simulink model "GPI1"  (Simulink 7.0)
settings: Solver=ode45  StartTime=0.0  StopTime=1000.0  RelTol=1e-3
values from neighbouring files (symbols this model uses):
  A_gpegpi = 1    [data_GPE.m]    (also in data_GPI.m)
  A_gpi = 2    [data_GPI.m]
  A_stngpi = 1    [data_GPI.m]    (also in data_STN.m)
  B_gpegpi = .1    (= 0.1)    [data_GPE.m]    (also in data_GPI.m)
  B_gpi = .08    (= 0.08)    [data_GPI.m]
  B_stngpi = .05    (= 0.05)    [data_GPI.m]    (also in data_STN.m)
  c_gpi = 1    [data_GPI.m]
  cagi0 = i_v_16(289:304)    [launch_sysGPI_mod.m]
  egpegpi = -100    [data_synapses.m]
  ek_gpi = -80.0    (= -80)    [data_GPI.m]
  el_gpi = -55.0    (= -55)    [data_GPI.m]
  epsil_gpi = 1*10^-4    (= 0.0001)    [data_GPI.m]
  estngpi = 0    [data_synapses.m]
  gahp_gpi = 30.0    (= 30)    [data_GPI.m]
  gca_gpi = 0.15    [data_GPI.m]
  ggpegpi = ggpegpi_vec(i)    [CN_launch_CN_analyze_TAL2.m]    (also in data_synapses.m = 1; launch_sysGPI_mod.m = 0.3)
  gk_gpi = 30.0    (= 30)    [data_GPI.m]
  gl_gpi = .1    (= 0.1)    [data_GPI.m]
  gna_gpi = 120    [data_GPI.m]
  gstngpi = .3    (= 0.3)    [data_synapses.m]
  gt_gpi = .5    (= 0.5)    [data_GPI.m]
  hgi0 = i_v_16(241:256)    [launch_sysGPI_mod.m]
  k1_gpi = 30.0    (= 30)    [data_GPI.m]
  kca_gpi = 15    [data_GPI.m]
  ngi0 = i_v_16(257:272)    [launch_sysGPI_mod.m]
  phih_gpi = 0.05    [data_GPI.m]
  phin_gpi = 0.1    [data_GPI.m]
  phir_gpi = 1    [data_GPI.m]
  rgi0 = i_v_16(273:288)    [launch_sysGPI_mod.m]
  sgi0 = i_v_16(305:320)    [launch_sysGPI_mod.m]
  sig0 = i_v_16(209:224)    [launch_sysGPI_mod.m]
  sigmaa_gpi = 2    [data_GPI.m]
  sigmagh_gpe = 2.0    (= 2)    [data_GPE.m]
  sigmagh_gpi = 2.0    (= 2)    [data_GPI.m]
  sigmagh_stn = 8.0    (= 8)    [data_STN.m]
  sigmah_gpi = -12    [data_GPI.m]
  sigmam_gpi = 10.0    (= 10)    [data_GPI.m]
  sigman_gpi = 14.0    (= 14)    [data_GPI.m]
  sigmar_gpi = -2.0    (= -2)    [data_GPI.m]
  sigmas_gpi = 2    [data_GPI.m]
  sigmatauh_gpi = -12    [data_GPI.m]
  sigmataun_gpi = -12.0    (= -12)    [data_GPI.m]
  sis0 = i_v_16(97:112)    [launch_sysGPI_mod.m]
  tauh0_gpi = .05    (= 0.05)    [data_GPI.m]
  tauh1_gpi = .27    (= 0.27)    [data_GPI.m]
  taun0_gpi = .05    (= 0.05)    [data_GPI.m]
  taun1_gpi = .27    (= 0.27)    [data_GPI.m]
  taur_gpi = 30.0    (= 30)    [data_GPI.m]
  theta_gpe = 20    [data_GPE.m]    (also in data_GPI.m)
  theta_gpi = 20    [data_GPI.m]
  theta_stn = 30    [data_GPI.m]    (also in data_STN.m)
  thetaa_gpi = -57.0    (= -57)    [data_GPI.m]
  thetagh_gpe = -57.0    (= -57)    [data_GPE.m]
  thetagh_gpi = -57.0    (= -57)    [data_GPI.m]
  thetagh_stn = -39.0    (= -39)    [data_STN.m]
  thetah_gpi = -58.0    (= -58)    [data_GPI.m]
  thetam_gpi = -37.0    (= -37)    [data_GPI.m]
  thetan_gpi = -50.0    (= -50)    [data_GPI.m]
  thetar_gpi = -70.0    (= -70)    [data_GPI.m]
  thetas_gpi = -35.0    (= -35)    [data_GPI.m]
  thetatauh_gpi = -40.0    (= -40)    [data_GPI.m]
  thetataun_gpi = -40.0    (= -40)    [data_GPI.m]
  vgi0 = i_v_16(225:240)    [launch_sysGPI_mod.m]
(part 1 of 6)
settings Model: Creator=marco  LastModifiedBy=marco  ExtModeAutoUpdateStatusClock=off
settings DataIOCC: ExternalInput=[t1,u1]  LoadExternalInput=on  SaveOutput=off  SignalLogging=off  SaveTime=off  SignalLoggingName=sigsOut
settings OptimizationCC: BooleanDataType=off
settings DebuggingCC: SaveWithParameterizedLinksMsg=none  SignalResolutionControl=TryResolveAllWithWarning  SolverPrmCheckMsg=none  MultiTaskDSMMsg=warning  MultiTaskCondExecSysMsg=none  StrictBusMsg=None
settings HardwareCC: TargetUnknown=on
settings RTWCC: IncludeERTFirstTime=on
settings GRTTargetCC: TargetFcnLib=ansi_tfl_tmw.mat

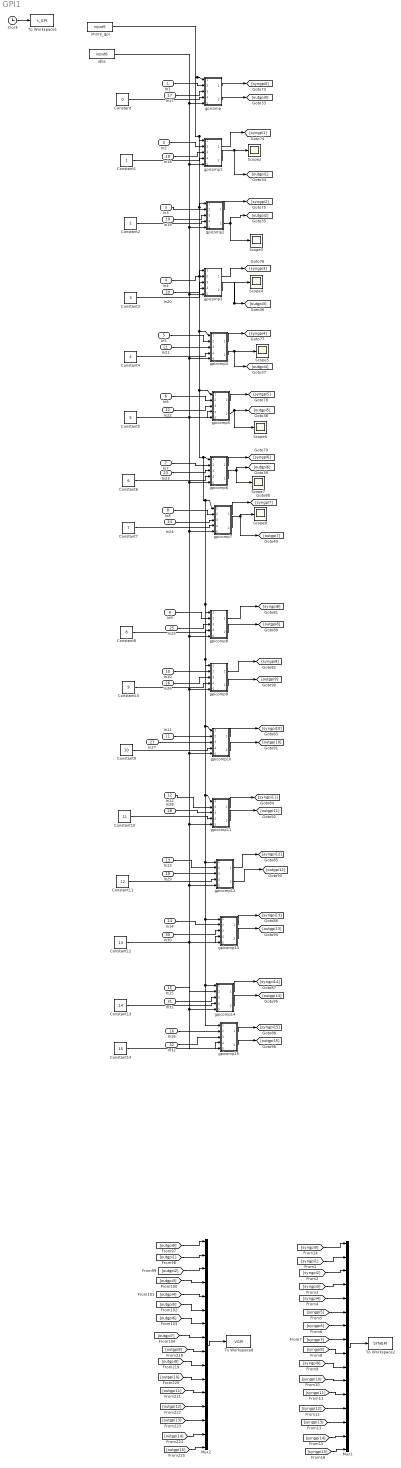
== system GPI1 ==
  In1 : Inport  OutDataType=sfix(16)  OutScaling=2^0
  In2 : Inport  Port=2  OutDataType=sfix(16)  OutScaling=2^0
  In3 : Inport  Port=3  OutDataType=sfix(16)  OutScaling=2^0
  In4 : Inport  Port=4  OutDataType=sfix(16)  OutScaling=2^0
  In5 : Inport  Port=5  OutDataType=sfix(16)  OutScaling=2^0
  In6 : Inport  Port=6  OutDataType=sfix(16)  OutScaling=2^0
  In7 : Inport  Port=7  OutDataType=sfix(16)  OutScaling=2^0
  In8 : Inport  Port=8  OutDataType=sfix(16)  OutScaling=2^0
  In9 : Inport  Port=9  OutDataType=sfix(16)  OutScaling=2^0
  In10 : Inport  Port=10  OutDataType=sfix(16)  OutScaling=2^0
  In11 : Inport  Port=11  OutDataType=sfix(16)  OutScaling=2^0
  In12 : Inport  Port=12  OutDataType=sfix(16)  OutScaling=2^0
  In13 : Inport  Port=13  OutDataType=sfix(16)  OutScaling=2^0
  In14 : Inport  Port=14  OutDataType=sfix(16)  OutScaling=2^0
  In15 : Inport  Port=15  OutDataType=sfix(16)  OutScaling=2^0
  In16 : Inport  Port=16  OutDataType=sfix(16)  OutScaling=2^0
  In17 : Inport  Port=17  OutDataType=sfix(16)  OutScaling=2^0
  In18 : Inport  Port=18  OutDataType=sfix(16)  OutScaling=2^0
  In19 : Inport  Port=19  OutDataType=sfix(16)  OutScaling=2^0
  In20 : Inport  Port=20  OutDataType=sfix(16)  OutScaling=2^0
  In21 : Inport  Port=21  OutDataType=sfix(16)  OutScaling=2^0
  In22 : Inport  Port=22  OutDataType=sfix(16)  OutScaling=2^0
  In23 : Inport  Port=23  OutDataType=sfix(16)  OutScaling=2^0
  In24 : Inport  Port=24  OutDataType=sfix(16)  OutScaling=2^0
  In25 : Inport  Port=25  OutDataType=sfix(16)  OutScaling=2^0
  In26 : Inport  Port=26  OutDataType=sfix(16)  OutScaling=2^0
  In27 : Inport  Port=27  OutDataType=sfix(16)  OutScaling=2^0
  In28 : Inport  Port=28  OutDataType=sfix(16)  OutScaling=2^0
  In29 : Inport  Port=29  OutDataType=sfix(16)  OutScaling=2^0
  In30 : Inport  Port=30  OutDataType=sfix(16)  OutScaling=2^0
  In31 : Inport  Port=31  OutDataType=sfix(16)  OutScaling=2^0
  In32 : Inport  Port=32  OutDataType=sfix(16)  OutScaling=2^0
  Clock : Clock
      settings: Decimation=10
  Constant : Constant  Value=0  OutDataType=sfix(16)  OutScaling=2^0
  Constant1 : Constant  OutDataType=sfix(16)  OutScaling=2^0
  Constant10 : Constant  Value=11  OutDataType=sfix(16)  OutScaling=2^0
  Constant11 : Constant  Value=12  OutDataType=sfix(16)  OutScaling=2^0
  Constant12 : Constant  Value=13  OutDataType=sfix(16)  OutScaling=2^0
  Constant13 : Constant  Value=14  OutDataType=sfix(16)  OutScaling=2^0
  Constant14 : Constant  Value=15  OutDataType=sfix(16)  OutScaling=2^0
  Constant15 : Constant  Value=9  OutDataType=sfix(16)  OutScaling=2^0
  Constant2 : Constant  Value=2  OutDataType=sfix(16)  OutScaling=2^0
  Constant3 : Constant  Value=3  OutDataType=sfix(16)  OutScaling=2^0
  Constant4 : Constant  Value=4  OutDataType=sfix(16)  OutScaling=2^0
  Constant5 : Constant  Value=5  OutDataType=sfix(16)  OutScaling=2^0
  Constant6 : Constant  Value=6  OutDataType=sfix(16)  OutScaling=2^0
  Constant7 : Constant  Value=7  OutDataType=sfix(16)  OutScaling=2^0
  Constant8 : Constant  Value=8  OutDataType=sfix(16)  OutScaling=2^0
  Constant9 : Constant  Value=10  OutDataType=sfix(16)  OutScaling=2^0
  Mux1 : Mux  Inputs=16
  Mux2 : Mux  Inputs=16
  Scope{2..8} (7 alike) : Scope
      Scope2 settings: YMin=-90  YMax=60  SaveName=ScopeData2
      Scope3 settings: YMin=-90  YMax=60  SaveName=ScopeData3
      Scope4 settings: YMin=-90  YMax=60  SaveName=ScopeData4
      Scope5 settings: SaveName=ScopeData5
      Scope6 settings: YMin=-90  YMax=60  SaveName=ScopeData6
      Scope7 settings: SaveName=ScopeData7
      Scope8 settings: YMin=-90  YMax=60  SaveName=ScopeData8
  To Workspace1 : ToWorkspace  VariableName=t_GPI  SampleTime=-1  SaveFormat=Array
  To Workspace2 : ToWorkspace  VariableName=SYNGPI  SampleTime=-1  SaveFormat=Array
  To Workspace8 : ToWorkspace  VariableName=VGPI  SampleTime=-1  SaveFormat=Array
  gpicomp : Subsystem
  gpicomp1 : Subsystem
  gpicomp10 : Subsystem
  gpicomp11 : Subsystem
  gpicomp12 : Subsystem
  gpicomp13 : Subsystem
  gpicomp14 : Subsystem
  gpicomp15 : Subsystem
  gpicomp2 : Subsystem
  gpicomp3 : Subsystem
  gpicomp4 : Subsystem
  gpicomp5 : Subsystem
  gpicomp6 : Subsystem
  gpicomp7 : Subsystem
  gpicomp8 : Subsystem
  gpicomp9 : Subsystem
  idbs : FromWorkspace  VariableName=input6  SampleTime=0.01
  imore_gpi : FromWorkspace  VariableName=input5  SampleTime=1
  wires:
  Clock/1 -> To Workspace1/1
  gpicomp6/2(Out2) -> Scope7/1, [outgpi6]
  gpicomp5/2(Out2) -> Scope6/1, [outgpi5]
  gpicomp4/2(Out2) -> Scope5/1, [outgpi4]
  gpicomp3/2(Out2) -> Scope4/1, [outgpi3]
  gpicomp/2(Out2) -> [outgpi0]
  gpicomp2/2(Out2) -> Scope3/1, [outgpi2]
  gpicomp1/2(Out2) -> Scope2/1, [outgpi1]
  imore_gpi/1 -> gpicomp/1(In1), gpicomp14/1(In1), gpicomp15/1(In1), gpicomp13/1(In1), gpicomp12/1(In1), gpicomp11/1(In1), gpicomp10/1(In1), gpicomp9/1(In1), gpicomp8/1(In1), gpicomp7/1(In1), gpicomp6/1(In1), gpicomp5/1(In1), gpicomp4/1(In1), gpicomp3/1(In1), gpicomp2/1(In1), gpicomp1/1(In1)
  gpicomp7/2(Out2) -> Scope8/1, [outgpi7]
  [outgpi0] -> Mux2/1
  [outgpi1] -> Mux2/2
  [outgpi2] -> Mux2/3
  [outgpi3] -> Mux2/4
  [outgpi4] -> Mux2/5
  [outgpi5] -> Mux2/6
  [outgpi6] -> Mux2/7
  [outgpi7] -> Mux2/8
  Mux2/1 -> To Workspace8/1
  gpicomp/1(Out1) -> [syngpi0]
  gpicomp1/1(Out1) -> [syngpi1]
  gpicomp2/1(Out1) -> [syngpi2]
  gpicomp3/1(Out1) -> [syngpi3]
  gpicomp4/1(Out1) -> [syngpi4]
  gpicomp5/1(Out1) -> [syngpi5]
  gpicomp6/1(Out1) -> [syngpi6]
  gpicomp7/1(Out1) -> [syngpi7]
  gpicomp8/1(Out1) -> [syngpi8]
  gpicomp9/1(Out1) -> [syngpi9]
  gpicomp10/1(Out1) -> [syngpi10]
  gpicomp11/1(Out1) -> [syngpi11]
  gpicomp12/1(Out1) -> [syngpi12]
  gpicomp13/1(Out1) -> [syngpi13]
  gpicomp14/1(Out1) -> [syngpi14]
  gpicomp15/1(Out1) -> [syngpi15]
  gpicomp13/2(Out2) -> [outgpi13]
  gpicomp14/2(Out2) -> [outgpi14]
  gpicomp15/2(Out2) -> [outgpi15]
  gpicomp12/2(Out2) -> [outgpi12]
  gpicomp11/2(Out2) -> [outgpi11]
  gpicomp10/2(Out2) -> [outgpi10]
  gpicomp9/2(Out2) -> [outgpi9]
  gpicomp8/2(Out2) -> [outgpi8]
  [outgpi8] -> Mux2/9
  [outgpi9] -> Mux2/10
  [outgpi10] -> Mux2/11
  [outgpi11] -> Mux2/12
  [outgpi12] -> Mux2/13
  [outgpi13] -> Mux2/14
  [outgpi14] -> Mux2/15
  [outgpi15] -> Mux2/16
  Constant14/1 -> gpicomp15/4(In4)
  Constant13/1 -> gpicomp14/4(In4)
  Constant12/1 -> gpicomp13/4(In4)
  Constant11/1 -> gpicomp12/4(In4)
  Constant10/1 -> gpicomp11/4(In4)
  Constant9/1 -> gpicomp10/4(In4)
  Constant15/1 -> gpicomp9/4(In4)
  Constant8/1 -> gpicomp8/4(In4)
  Constant7/1 -> gpicomp7/4(In4)
  Constant6/1 -> gpicomp6/4(In4)
  Constant5/1 -> gpicomp5/4(In4)
  Constant4/1 -> gpicomp4/4(In4)
  Constant3/1 -> gpicomp3/4(In4)
  Constant2/1 -> gpicomp2/4(In4)
  Constant1/1 -> gpicomp1/4(In4)
  Constant/1 -> gpicomp/4(In4)
  In1/1 -> gpicomp/2(In2)
  In2/1 -> gpicomp1/2(In2)
  In3/1 -> gpicomp2/2(In2)
  In4/1 -> gpicomp3/2(In2)
  In5/1 -> gpicomp4/2(In2)
  In6/1 -> gpicomp5/2(In2)
  In7/1 -> gpicomp6/2(In2)
  In8/1 -> gpicomp7/2(In2)
  In9/1 -> gpicomp8/2(In2)
  In10/1 -> gpicomp9/2(In2)
  In11/1 -> gpicomp10/2(In2)
  In12/1 -> gpicomp11/2(In2)
  In13/1 -> gpicomp12/2(In2)
  In14/1 -> gpicomp13/2(In2)
  In15/1 -> gpicomp14/2(In2)
  In16/1 -> gpicomp15/2(In2)
  In32/1 -> gpicomp15/3(In3)
  In31/1 -> gpicomp14/3(In3)
  In30/1 -> gpicomp13/3(In3)
  In29/1 -> gpicomp12/3(In3)
  In28/1 -> gpicomp11/3(In3)
  In27/1 -> gpicomp10/3(In3)
  In26/1 -> gpicomp9/3(In3)
  In25/1 -> gpicomp8/3(In3)
  In24/1 -> gpicomp7/3(In3)
  In23/1 -> gpicomp6/3(In3)
  In22/1 -> gpicomp5/3(In3)
  In21/1 -> gpicomp4/3(In3)
  In20/1 -> gpicomp3/3(In3)
  In19/1 -> gpicomp2/3(In3)
  In18/1 -> gpicomp1/3(In3)
  In17/1 -> gpicomp/3(In3)
  [syngpi0] -> Mux1/1
  [syngpi2] -> Mux1/3
  Mux1/1 -> To Workspace2/1
  [syngpi8] -> Mux1/9
  [syngpi9] -> Mux1/10
  [syngpi10] -> Mux1/11
  [syngpi11] -> Mux1/12
  [syngpi12] -> Mux1/13
  [syngpi13] -> Mux1/14
  [syngpi14] -> Mux1/15
  [syngpi15] -> Mux1/16
  [syngpi1] -> Mux1/2
  [syngpi3] -> Mux1/4
  [syngpi4] -> Mux1/5
  [syngpi5] -> Mux1/6
  [syngpi6] -> Mux1/7
  [syngpi7] -> Mux1/8
  idbs/1 -> gpicomp/5(In5), gpicomp1/5(In5), gpicomp2/5(In5), gpicomp3/5(In5), gpicomp4/5(In5), gpicomp6/5(In5), gpicomp7/5(In5), gpicomp8/5(In5), gpicomp9/5(In5), gpicomp10/5(In5), gpicomp11/5(In5), gpicomp12/5(In5), gpicomp14/5(In5), gpicomp15/5(In5), gpicomp13/5(In5), gpicomp5/5(In5)

== system GPI1/gpicomp ==
  In1 : Inport  OutDataType=sfix(16)  OutScaling=2^0
  In2 : Inport  Port=2  OutDataType=sfix(16)  OutScaling=2^0
  In3 : Inport  Port=3  OutDataType=sfix(16)  OutScaling=2^0
  In4 : Inport  Port=4  OutDataType=sfix(16)  OutScaling=2^0
  In5 : Inport  Port=5  OutDataType=sfix(16)  OutScaling=2^0
  Constant : Constant  Value=sis0  OutDataType=sfix(16)  OutScaling=2^0
  Constant1 : Constant  Value=sig0  OutDataType=sfix(16)  OutScaling=2^0
  Constant2 : Constant  Value=sgi0  OutDataType=sfix(16)  OutScaling=2^0
  Selector1 : Selector  IndexMode=Zero-based  IndexOptions=Index vector (port)  Indices=[1 3]  OutputSizes=1
  Selector2 : Selector  IndexMode=Zero-based  IndexOptions=Index vector (port)  Indices=[1 3]  OutputSizes=1
  Selector5 : Selector  IndexMode=Zero-based  IndexOptions=Index vector (port)  Indices=[1 3]  OutputSizes=1
  gpi_cell : Subsystem
  igpegpi : Subsystem
  istngpi : Subsystem
  syn_gpegpi : Subsystem
  syn_gpegpi1 : Subsystem
  syn_stngpi : Subsystem
  Out1 : Outport  OutDataType=sfix(16)  OutScaling=2^0
  Out2 : Outport  Port=2  OutDataType=sfix(16)  OutScaling=2^0
  wires:
  igpegpi/1(Out1) -> gpi_cell/3(In3)
  istngpi/1(Out1) -> gpi_cell/2(In2)
  syn_gpegpi/1(Out1) -> igpegpi/1(In1)
  syn_stngpi/1(Out1) -> istngpi/1(In1)
  syn_gpegpi1/1(Out1) -> Out1/1
  In1/1 -> gpi_cell/1(In1)
  In2/1 -> syn_stngpi/1(In1)
  In3/1 -> syn_gpegpi/1(In1)
  gpi_cell/1(Out1) -> Out2/1, istngpi/2(In3), igpegpi/2(In3), syn_gpegpi1/1(In1)
  Selector2/1 -> syn_gpegpi1/2(In2)
  In4/1 -> Selector5/2, Selector2/2, gpi_cell/4(In4), Selector1/2
  Selector5/1 -> syn_stngpi/2(In2)
  Selector1/1 -> syn_gpegpi/2(In2)
  Constant2/1 -> Selector2/1
  Constant/1 -> Selector5/1
  Constant1/1 -> Selector1/1
  In5/1 -> gpi_cell/5(In5)

== system GPI1/gpicomp1 ==
  In1 : Inport  OutDataType=sfix(16)  OutScaling=2^0
  In2 : Inport  Port=2  OutDataType=sfix(16)  OutScaling=2^0
  In3 : Inport  Port=3  OutDataType=sfix(16)  OutScaling=2^0
  In4 : Inport  Port=4  OutDataType=sfix(16)  OutScaling=2^0
  In5 : Inport  Port=5  OutDataType=sfix(16)  OutScaling=2^0
  Constant : Constant  Value=sis0  OutDataType=sfix(16)  OutScaling=2^0
  Constant1 : Constant  Value=sig0  OutDataType=sfix(16)  OutScaling=2^0
  Constant2 : Constant  Value=sgi0  OutDataType=sfix(16)  OutScaling=2^0
  Selector1 : Selector  IndexMode=Zero-based  IndexOptions=Index vector (port)  Indices=[1 3]  OutputSizes=1
  Selector2 : Selector  IndexMode=Zero-based  IndexOptions=Index vector (port)  Indices=[1 3]  OutputSizes=1
  Selector5 : Selector  IndexMode=Zero-based  IndexOptions=Index vector (port)  Indices=[1 3]  OutputSizes=1
  gpi_cell : Subsystem
  igpegpi : Subsystem
  istngpi : Subsystem
  syn_gpegpi : Subsystem
  syn_gpegpi1 : Subsystem
  syn_stngpi : Subsystem
  Out1 : Outport  OutDataType=sfix(16)  OutScaling=2^0
  Out2 : Outport  Port=2  OutDataType=sfix(16)  OutScaling=2^0
  wires:
  igpegpi/1(Out1) -> gpi_cell/3(In3)
  istngpi/1(Out1) -> gpi_cell/2(In2)
  syn_gpegpi/1(Out1) -> igpegpi/1(In1)
  syn_stngpi/1(Out1) -> istngpi/1(In1)
  syn_gpegpi1/1(Out1) -> Out1/1
  In1/1 -> gpi_cell/1(In1)
  In2/1 -> syn_stngpi/1(In1)
  In3/1 -> syn_gpegpi/1(In1)
  gpi_cell/1(Out1) -> Out2/1, istngpi/2(In3), igpegpi/2(In3), syn_gpegpi1/1(In1)
  Selector2/1 -> syn_gpegpi1/2(In2)
  In4/1 -> Selector5/2, Selector2/2, gpi_cell/4(In4), Selector1/2
  Selector5/1 -> syn_stngpi/2(In2)
  Selector1/1 -> syn_gpegpi/2(In2)
  Constant2/1 -> Selector2/1
  Constant/1 -> Selector5/1
  Constant1/1 -> Selector1/1
  In5/1 -> gpi_cell/5(In5)

== system GPI1/gpicomp10 ==
  In1 : Inport  OutDataType=sfix(16)  OutScaling=2^0
  In2 : Inport  Port=2  OutDataType=sfix(16)  OutScaling=2^0
  In3 : Inport  Port=3  OutDataType=sfix(16)  OutScaling=2^0
  In4 : Inport  Port=4  OutDataType=sfix(16)  OutScaling=2^0
  In5 : Inport  Port=5  OutDataType=sfix(16)  OutScaling=2^0
  Constant : Constant  Value=sis0  OutDataType=sfix(16)  OutScaling=2^0
  Constant1 : Constant  Value=sig0  OutDataType=sfix(16)  OutScaling=2^0
  Constant2 : Constant  Value=sgi0  OutDataType=sfix(16)  OutScaling=2^0
  Selector1 : Selector  IndexMode=Zero-based  IndexOptions=Index vector (port)  Indices=[1 3]  OutputSizes=1
  Selector2 : Selector  IndexMode=Zero-based  IndexOptions=Index vector (port)  Indices=[1 3]  OutputSizes=1
  Selector5 : Selector  IndexMode=Zero-based  IndexOptions=Index vector (port)  Indices=[1 3]  OutputSizes=1
  gpi_cell : Subsystem
  igpegpi : Subsystem
  istngpi : Subsystem
  syn_gpegpi : Subsystem
  syn_gpegpi1 : Subsystem
  syn_stngpi : Subsystem
  Out1 : Outport  OutDataType=sfix(16)  OutScaling=2^0
  Out2 : Outport  Port=2  OutDataType=sfix(16)  OutScaling=2^0
  wires:
  igpegpi/1(Out1) -> gpi_cell/3(In3)
  istngpi/1(Out1) -> gpi_cell/2(In2)
  syn_gpegpi/1(Out1) -> igpegpi/1(In1)
  syn_stngpi/1(Out1) -> istngpi/1(In1)
  syn_gpegpi1/1(Out1) -> Out1/1
  In1/1 -> gpi_cell/1(In1)
  In2/1 -> syn_stngpi/1(In1)
  In3/1 -> syn_gpegpi/1(In1)
  gpi_cell/1(Out1) -> Out2/1, istngpi/2(In3), igpegpi/2(In3), syn_gpegpi1/1(In1)
  Selector2/1 -> syn_gpegpi1/2(In2)
  In4/1 -> Selector5/2, Selector2/2, gpi_cell/4(In4), Selector1/2
  Selector5/1 -> syn_stngpi/2(In2)
  Selector1/1 -> syn_gpegpi/2(In2)
  Constant2/1 -> Selector2/1
  Constant/1 -> Selector5/1
  Constant1/1 -> Selector1/1
  In5/1 -> gpi_cell/5(In5)

== system GPI1/gpicomp11 ==
  In1 : Inport  OutDataType=sfix(16)  OutScaling=2^0
  In2 : Inport  Port=2  OutDataType=sfix(16)  OutScaling=2^0
  In3 : Inport  Port=3  OutDataType=sfix(16)  OutScaling=2^0
  In4 : Inport  Port=4  OutDataType=sfix(16)  OutScaling=2^0
  In5 : Inport  Port=5  OutDataType=sfix(16)  OutScaling=2^0
  Constant : Constant  Value=sis0  OutDataType=sfix(16)  OutScaling=2^0
  Constant1 : Constant  Value=sig0  OutDataType=sfix(16)  OutScaling=2^0
  Constant2 : Constant  Value=sgi0  OutDataType=sfix(16)  OutScaling=2^0
  Selector1 : Selector  IndexMode=Zero-based  IndexOptions=Index vector (port)  Indices=[1 3]  OutputSizes=1
  Selector2 : Selector  IndexMode=Zero-based  IndexOptions=Index vector (port)  Indices=[1 3]  OutputSizes=1
  Selector5 : Selector  IndexMode=Zero-based  IndexOptions=Index vector (port)  Indices=[1 3]  OutputSizes=1
  gpi_cell : Subsystem
  igpegpi : Subsystem
  istngpi : Subsystem
  syn_gpegpi : Subsystem
  syn_gpegpi1 : Subsystem
  syn_stngpi : Subsystem
  Out1 : Outport  OutDataType=sfix(16)  OutScaling=2^0
  Out2 : Outport  Port=2  OutDataType=sfix(16)  OutScaling=2^0
  wires:
  igpegpi/1(Out1) -> gpi_cell/3(In3)
  istngpi/1(Out1) -> gpi_cell/2(In2)
  syn_gpegpi/1(Out1) -> igpegpi/1(In1)
  syn_stngpi/1(Out1) -> istngpi/1(In1)
  syn_gpegpi1/1(Out1) -> Out1/1
  In1/1 -> gpi_cell/1(In1)
  In2/1 -> syn_stngpi/1(In1)
  In3/1 -> syn_gpegpi/1(In1)
  gpi_cell/1(Out1) -> Out2/1, istngpi/2(In3), igpegpi/2(In3), syn_gpegpi1/1(In1)
  Selector2/1 -> syn_gpegpi1/2(In2)
  In4/1 -> Selector5/2, Selector2/2, gpi_cell/4(In4), Selector1/2
  Selector5/1 -> syn_stngpi/2(In2)
  Selector1/1 -> syn_gpegpi/2(In2)
  Constant2/1 -> Selector2/1
  Constant/1 -> Selector5/1
  Constant1/1 -> Selector1/1
  In5/1 -> gpi_cell/5(In5)

== system GPI1/gpicomp12 ==
  In1 : Inport  OutDataType=sfix(16)  OutScaling=2^0
  In2 : Inport  Port=2  OutDataType=sfix(16)  OutScaling=2^0
  In3 : Inport  Port=3  OutDataType=sfix(16)  OutScaling=2^0
  In4 : Inport  Port=4  OutDataType=sfix(16)  OutScaling=2^0
  In5 : Inport  Port=5  OutDataType=sfix(16)  OutScaling=2^0
  Constant : Constant  Value=sis0  OutDataType=sfix(16)  OutScaling=2^0
  Constant1 : Constant  Value=sig0  OutDataType=sfix(16)  OutScaling=2^0
  Constant2 : Constant  Value=sgi0  OutDataType=sfix(16)  OutScaling=2^0
  Selector1 : Selector  IndexMode=Zero-based  IndexOptions=Index vector (port)  Indices=[1 3]  OutputSizes=1
  Selector2 : Selector  IndexMode=Zero-based  IndexOptions=Index vector (port)  Indices=[1 3]  OutputSizes=1
  Selector5 : Selector  IndexMode=Zero-based  IndexOptions=Index vector (port)  Indices=[1 3]  OutputSizes=1
  gpi_cell : Subsystem
  igpegpi : Subsystem
  istngpi : Subsystem
  syn_gpegpi : Subsystem
  syn_gpegpi1 : Subsystem
  syn_stngpi : Subsystem
  Out1 : Outport  OutDataType=sfix(16)  OutScaling=2^0
  Out2 : Outport  Port=2  OutDataType=sfix(16)  OutScaling=2^0
  wires:
  igpegpi/1(Out1) -> gpi_cell/3(In3)
  istngpi/1(Out1) -> gpi_cell/2(In2)
  syn_gpegpi/1(Out1) -> igpegpi/1(In1)
  syn_stngpi/1(Out1) -> istngpi/1(In1)
  syn_gpegpi1/1(Out1) -> Out1/1
  In1/1 -> gpi_cell/1(In1)
  In2/1 -> syn_stngpi/1(In1)
  In3/1 -> syn_gpegpi/1(In1)
  gpi_cell/1(Out1) -> Out2/1, istngpi/2(In3), igpegpi/2(In3), syn_gpegpi1/1(In1)
  Selector2/1 -> syn_gpegpi1/2(In2)
  In4/1 -> Selector5/2, Selector2/2, gpi_cell/4(In4), Selector1/2
  Selector5/1 -> syn_stngpi/2(In2)
  Selector1/1 -> syn_gpegpi/2(In2)
  Constant2/1 -> Selector2/1
  Constant/1 -> Selector5/1
  Constant1/1 -> Selector1/1
  In5/1 -> gpi_cell/5(In5)

== system GPI1/gpicomp13 ==
  In1 : Inport  OutDataType=sfix(16)  OutScaling=2^0
  In2 : Inport  Port=2  OutDataType=sfix(16)  OutScaling=2^0
  In3 : Inport  Port=3  OutDataType=sfix(16)  OutScaling=2^0
  In4 : Inport  Port=4  OutDataType=sfix(16)  OutScaling=2^0
  In5 : Inport  Port=5  OutDataType=sfix(16)  OutScaling=2^0
  Constant : Constant  Value=sis0  OutDataType=sfix(16)  OutScaling=2^0
  Constant1 : Constant  Value=sig0  OutDataType=sfix(16)  OutScaling=2^0
  Constant2 : Constant  Value=sgi0  OutDataType=sfix(16)  OutScaling=2^0
  Selector1 : Selector  IndexMode=Zero-based  IndexOptions=Index vector (port)  Indices=[1 3]  OutputSizes=1
  Selector2 : Selector  IndexMode=Zero-based  IndexOptions=Index vector (port)  Indices=[1 3]  OutputSizes=1
  Selector5 : Selector  IndexMode=Zero-based  IndexOptions=Index vector (port)  Indices=[1 3]  OutputSizes=1
  gpi_cell : Subsystem
  igpegpi : Subsystem
  istngpi : Subsystem
  syn_gpegpi : Subsystem
  syn_gpegpi1 : Subsystem
  syn_stngpi : Subsystem
  Out1 : Outport  OutDataType=sfix(16)  OutScaling=2^0
  Out2 : Outport  Port=2  OutDataType=sfix(16)  OutScaling=2^0
  wires:
  igpegpi/1(Out1) -> gpi_cell/3(In3)
  istngpi/1(Out1) -> gpi_cell/2(In2)
  syn_gpegpi/1(Out1) -> igpegpi/1(In1)
  syn_stngpi/1(Out1) -> istngpi/1(In1)
  syn_gpegpi1/1(Out1) -> Out1/1
  In1/1 -> gpi_cell/1(In1)
  In2/1 -> syn_stngpi/1(In1)
  In3/1 -> syn_gpegpi/1(In1)
  gpi_cell/1(Out1) -> Out2/1, istngpi/2(In3), igpegpi/2(In3), syn_gpegpi1/1(In1)
  Selector2/1 -> syn_gpegpi1/2(In2)
  In4/1 -> Selector5/2, Selector2/2, gpi_cell/4(In4), Selector1/2
  Selector5/1 -> syn_stngpi/2(In2)
  Selector1/1 -> syn_gpegpi/2(In2)
  Constant2/1 -> Selector2/1
  Constant/1 -> Selector5/1
  Constant1/1 -> Selector1/1
  In5/1 -> gpi_cell/5(In5)

== system GPI1/gpicomp14 ==
  In1 : Inport  OutDataType=sfix(16)  OutScaling=2^0
  In2 : Inport  Port=2  OutDataType=sfix(16)  OutScaling=2^0
  In3 : Inport  Port=3  OutDataType=sfix(16)  OutScaling=2^0
  In4 : Inport  Port=4  OutDataType=sfix(16)  OutScaling=2^0
  In5 : Inport  Port=5  OutDataType=sfix(16)  OutScaling=2^0
  Constant : Constant  Value=sis0  OutDataType=sfix(16)  OutScaling=2^0
  Constant1 : Constant  Value=sig0  OutDataType=sfix(16)  OutScaling=2^0
  Constant2 : Constant  Value=sgi0  OutDataType=sfix(16)  OutScaling=2^0
  Selector1 : Selector  IndexMode=Zero-based  IndexOptions=Index vector (port)  Indices=[1 3]  OutputSizes=1
  Selector2 : Selector  IndexMode=Zero-based  IndexOptions=Index vector (port)  Indices=[1 3]  OutputSizes=1
  Selector5 : Selector  IndexMode=Zero-based  IndexOptions=Index vector (port)  Indices=[1 3]  OutputSizes=1
  gpi_cell : Subsystem
  igpegpi : Subsystem
  istngpi : Subsystem
  syn_gpegpi : Subsystem
  syn_gpegpi1 : Subsystem
  syn_stngpi : Subsystem
  Out1 : Outport  OutDataType=sfix(16)  OutScaling=2^0
  Out2 : Outport  Port=2  OutDataType=sfix(16)  OutScaling=2^0
  wires:
  igpegpi/1(Out1) -> gpi_cell/3(In3)
  istngpi/1(Out1) -> gpi_cell/2(In2)
  syn_gpegpi/1(Out1) -> igpegpi/1(In1)
  syn_stngpi/1(Out1) -> istngpi/1(In1)
  syn_gpegpi1/1(Out1) -> Out1/1
  In1/1 -> gpi_cell/1(In1)
  In2/1 -> syn_stngpi/1(In1)
  In3/1 -> syn_gpegpi/1(In1)
  gpi_cell/1(Out1) -> Out2/1, istngpi/2(In3), igpegpi/2(In3), syn_gpegpi1/1(In1)
  Selector2/1 -> syn_gpegpi1/2(In2)
  In4/1 -> Selector5/2, Selector2/2, gpi_cell/4(In4), Selector1/2
  Selector5/1 -> syn_stngpi/2(In2)
  Selector1/1 -> syn_gpegpi/2(In2)
  Constant2/1 -> Selector2/1
  Constant/1 -> Selector5/1
  Constant1/1 -> Selector1/1
  In5/1 -> gpi_cell/5(In5)

== system GPI1/gpicomp15 ==
  In1 : Inport  OutDataType=sfix(16)  OutScaling=2^0
  In2 : Inport  Port=2  OutDataType=sfix(16)  OutScaling=2^0
  In3 : Inport  Port=3  OutDataType=sfix(16)  OutScaling=2^0
  In4 : Inport  Port=4  OutDataType=sfix(16)  OutScaling=2^0
  In5 : Inport  Port=5  OutDataType=sfix(16)  OutScaling=2^0
  Constant : Constant  Value=sis0  OutDataType=sfix(16)  OutScaling=2^0
  Constant1 : Constant  Value=sig0  OutDataType=sfix(16)  OutScaling=2^0
  Constant2 : Constant  Value=sgi0  OutDataType=sfix(16)  OutScaling=2^0
  Selector1 : Selector  IndexMode=Zero-based  IndexOptions=Index vector (port)  Indices=[1 3]  OutputSizes=1
  Selector2 : Selector  IndexMode=Zero-based  IndexOptions=Index vector (port)  Indices=[1 3]  OutputSizes=1
  Selector5 : Selector  IndexMode=Zero-based  IndexOptions=Index vector (port)  Indices=[1 3]  OutputSizes=1
  gpi_cell : Subsystem
  igpegpi : Subsystem
  istngpi : Subsystem
  syn_gpegpi : Subsystem
  syn_gpegpi1 : Subsystem
  syn_stngpi : Subsystem
  Out1 : Outport  OutDataType=sfix(16)  OutScaling=2^0
  Out2 : Outport  Port=2  OutDataType=sfix(16)  OutScaling=2^0
  wires:
  igpegpi/1(Out1) -> gpi_cell/3(In3)
  istngpi/1(Out1) -> gpi_cell/2(In2)
  syn_gpegpi/1(Out1) -> igpegpi/1(In1)
  syn_stngpi/1(Out1) -> istngpi/1(In1)
  syn_gpegpi1/1(Out1) -> Out1/1
  In1/1 -> gpi_cell/1(In1)
  In2/1 -> syn_stngpi/1(In1)
  In3/1 -> syn_gpegpi/1(In1)
  gpi_cell/1(Out1) -> Out2/1, istngpi/2(In3), igpegpi/2(In3), syn_gpegpi1/1(In1)
  Selector2/1 -> syn_gpegpi1/2(In2)
  In4/1 -> Selector5/2, Selector2/2, gpi_cell/4(In4), Selector1/2
  Selector5/1 -> syn_stngpi/2(In2)
  Selector1/1 -> syn_gpegpi/2(In2)
  Constant2/1 -> Selector2/1
  Constant/1 -> Selector5/1
  Constant1/1 -> Selector1/1
  In5/1 -> gpi_cell/5(In5)

== system GPI1/gpicomp2 ==
  In1 : Inport  OutDataType=sfix(16)  OutScaling=2^0
  In2 : Inport  Port=2  OutDataType=sfix(16)  OutScaling=2^0
  In3 : Inport  Port=3  OutDataType=sfix(16)  OutScaling=2^0
  In4 : Inport  Port=4  OutDataType=sfix(16)  OutScaling=2^0
  In5 : Inport  Port=5  OutDataType=sfix(16)  OutScaling=2^0
  Constant : Constant  Value=sis0  OutDataType=sfix(16)  OutScaling=2^0
  Constant1 : Constant  Value=sig0  OutDataType=sfix(16)  OutScaling=2^0
  Constant2 : Constant  Value=sgi0  OutDataType=sfix(16)  OutScaling=2^0
  Selector1 : Selector  IndexMode=Zero-based  IndexOptions=Index vector (port)  Indices=[1 3]  OutputSizes=1
  Selector2 : Selector  IndexMode=Zero-based  IndexOptions=Index vector (port)  Indices=[1 3]  OutputSizes=1
  Selector5 : Selector  IndexMode=Zero-based  IndexOptions=Index vector (port)  Indices=[1 3]  OutputSizes=1
  gpi_cell : Subsystem
  igpegpi : Subsystem
  istngpi : Subsystem
  syn_gpegpi : Subsystem
  syn_gpegpi1 : Subsystem
  syn_stngpi : Subsystem
  Out1 : Outport  OutDataType=sfix(16)  OutScaling=2^0
  Out2 : Outport  Port=2  OutDataType=sfix(16)  OutScaling=2^0
  wires:
  igpegpi/1(Out1) -> gpi_cell/3(In3)
  istngpi/1(Out1) -> gpi_cell/2(In2)
  syn_gpegpi/1(Out1) -> igpegpi/1(In1)
  syn_stngpi/1(Out1) -> istngpi/1(In1)
  syn_gpegpi1/1(Out1) -> Out1/1
  In1/1 -> gpi_cell/1(In1)
  In2/1 -> syn_stngpi/1(In1)
  In3/1 -> syn_gpegpi/1(In1)
  gpi_cell/1(Out1) -> Out2/1, istngpi/2(In3), igpegpi/2(In3), syn_gpegpi1/1(In1)
  Selector2/1 -> syn_gpegpi1/2(In2)
  In4/1 -> Selector5/2, Selector2/2, gpi_cell/4(In4), Selector1/2
  Selector5/1 -> syn_stngpi/2(In2)
  Selector1/1 -> syn_gpegpi/2(In2)
  Constant2/1 -> Selector2/1
  Constant/1 -> Selector5/1
  Constant1/1 -> Selector1/1
  In5/1 -> gpi_cell/5(In5)

== system GPI1/gpicomp3 ==
  In1 : Inport  OutDataType=sfix(16)  OutScaling=2^0
  In2 : Inport  Port=2  OutDataType=sfix(16)  OutScaling=2^0
  In3 : Inport  Port=3  OutDataType=sfix(16)  OutScaling=2^0
  In4 : Inport  Port=4  OutDataType=sfix(16)  OutScaling=2^0
  In5 : Inport  Port=5  OutDataType=sfix(16)  OutScaling=2^0
  Constant : Constant  Value=sis0  OutDataType=sfix(16)  OutScaling=2^0
  Constant1 : Constant  Value=sig0  OutDataType=sfix(16)  OutScaling=2^0
  Constant2 : Constant  Value=sgi0  OutDataType=sfix(16)  OutScaling=2^0
  Selector1 : Selector  IndexMode=Zero-based  IndexOptions=Index vector (port)  Indices=[1 3]  OutputSizes=1
  Selector2 : Selector  IndexMode=Zero-based  IndexOptions=Index vector (port)  Indices=[1 3]  OutputSizes=1
  Selector5 : Selector  IndexMode=Zero-based  IndexOptions=Index vector (port)  Indices=[1 3]  OutputSizes=1
  gpi_cell : Subsystem
  igpegpi : Subsystem
  istngpi : Subsystem
  syn_gpegpi : Subsystem
  syn_gpegpi1 : Subsystem
  syn_stngpi : Subsystem
  Out1 : Outport  OutDataType=sfix(16)  OutScaling=2^0
  Out2 : Outport  Port=2  OutDataType=sfix(16)  OutScaling=2^0
  wires:
  igpegpi/1(Out1) -> gpi_cell/3(In3)
  istngpi/1(Out1) -> gpi_cell/2(In2)
  syn_gpegpi/1(Out1) -> igpegpi/1(In1)
  syn_stngpi/1(Out1) -> istngpi/1(In1)
  syn_gpegpi1/1(Out1) -> Out1/1
  In1/1 -> gpi_cell/1(In1)
  In2/1 -> syn_stngpi/1(In1)
  In3/1 -> syn_gpegpi/1(In1)
  gpi_cell/1(Out1) -> Out2/1, istngpi/2(In3), igpegpi/2(In3), syn_gpegpi1/1(In1)
  Selector2/1 -> syn_gpegpi1/2(In2)
  In4/1 -> Selector5/2, Selector2/2, gpi_cell/4(In4), Selector1/2
  Selector5/1 -> syn_stngpi/2(In2)
  Selector1/1 -> syn_gpegpi/2(In2)
  Constant2/1 -> Selector2/1
  Constant/1 -> Selector5/1
  Constant1/1 -> Selector1/1
  In5/1 -> gpi_cell/5(In5)

== system GPI1/gpicomp4 ==
  In1 : Inport  OutDataType=sfix(16)  OutScaling=2^0
  In2 : Inport  Port=2  OutDataType=sfix(16)  OutScaling=2^0
  In3 : Inport  Port=3  OutDataType=sfix(16)  OutScaling=2^0
  In4 : Inport  Port=4  OutDataType=sfix(16)  OutScaling=2^0
  In5 : Inport  Port=5  OutDataType=sfix(16)  OutScaling=2^0
  Constant : Constant  Value=sis0  OutDataType=sfix(16)  OutScaling=2^0
  Constant1 : Constant  Value=sig0  OutDataType=sfix(16)  OutScaling=2^0
  Constant2 : Constant  Value=sgi0  OutDataType=sfix(16)  OutScaling=2^0
  Selector1 : Selector  IndexMode=Zero-based  IndexOptions=Index vector (port)  Indices=[1 3]  OutputSizes=1
  Selector2 : Selector  IndexMode=Zero-based  IndexOptions=Index vector (port)  Indices=[1 3]  OutputSizes=1
  Selector5 : Selector  IndexMode=Zero-based  IndexOptions=Index vector (port)  Indices=[1 3]  OutputSizes=1
  gpi_cell : Subsystem
  igpegpi : Subsystem
  istngpi : Subsystem
  syn_gpegpi : Subsystem
  syn_gpegpi1 : Subsystem
  syn_stngpi : Subsystem
  Out1 : Outport  OutDataType=sfix(16)  OutScaling=2^0
  Out2 : Outport  Port=2  OutDataType=sfix(16)  OutScaling=2^0
  wires:
  igpegpi/1(Out1) -> gpi_cell/3(In3)
  istngpi/1(Out1) -> gpi_cell/2(In2)
  syn_gpegpi/1(Out1) -> igpegpi/1(In1)
  syn_stngpi/1(Out1) -> istngpi/1(In1)
  syn_gpegpi1/1(Out1) -> Out1/1
  In1/1 -> gpi_cell/1(In1)
  In2/1 -> syn_stngpi/1(In1)
  In3/1 -> syn_gpegpi/1(In1)
  gpi_cell/1(Out1) -> Out2/1, istngpi/2(In3), igpegpi/2(In3), syn_gpegpi1/1(In1)
  Selector2/1 -> syn_gpegpi1/2(In2)
  In4/1 -> Selector5/2, Selector2/2, gpi_cell/4(In4), Selector1/2
  Selector5/1 -> syn_stngpi/2(In2)
  Selector1/1 -> syn_gpegpi/2(In2)
  Constant2/1 -> Selector2/1
  Constant/1 -> Selector5/1
  Constant1/1 -> Selector1/1
  In5/1 -> gpi_cell/5(In5)

== system GPI1/gpicomp5 ==
  In1 : Inport  OutDataType=sfix(16)  OutScaling=2^0
  In2 : Inport  Port=2  OutDataType=sfix(16)  OutScaling=2^0
  In3 : Inport  Port=3  OutDataType=sfix(16)  OutScaling=2^0
  In4 : Inport  Port=4  OutDataType=sfix(16)  OutScaling=2^0
  In5 : Inport  Port=5  OutDataType=sfix(16)  OutScaling=2^0
  Constant : Constant  Value=sis0  OutDataType=sfix(16)  OutScaling=2^0
  Constant1 : Constant  Value=sig0  OutDataType=sfix(16)  OutScaling=2^0
  Constant2 : Constant  Value=sgi0  OutDataType=sfix(16)  OutScaling=2^0
  Selector1 : Selector  IndexMode=Zero-based  IndexOptions=Index vector (port)  Indices=[1 3]  OutputSizes=1
  Selector2 : Selector  IndexMode=Zero-based  IndexOptions=Index vector (port)  Indices=[1 3]  OutputSizes=1
  Selector5 : Selector  IndexMode=Zero-based  IndexOptions=Index vector (port)  Indices=[1 3]  OutputSizes=1
  gpi_cell : Subsystem
  igpegpi : Subsystem
  istngpi : Subsystem
  syn_gpegpi : Subsystem
  syn_gpegpi1 : Subsystem
  syn_stngpi : Subsystem
  Out1 : Outport  OutDataType=sfix(16)  OutScaling=2^0
  Out2 : Outport  Port=2  OutDataType=sfix(16)  OutScaling=2^0
  wires:
  igpegpi/1(Out1) -> gpi_cell/3(In3)
  istngpi/1(Out1) -> gpi_cell/2(In2)
  syn_gpegpi/1(Out1) -> igpegpi/1(In1)
  syn_stngpi/1(Out1) -> istngpi/1(In1)
  syn_gpegpi1/1(Out1) -> Out1/1
  In1/1 -> gpi_cell/1(In1)
  In2/1 -> syn_stngpi/1(In1)
  In3/1 -> syn_gpegpi/1(In1)
  gpi_cell/1(Out1) -> Out2/1, istngpi/2(In3), igpegpi/2(In3), syn_gpegpi1/1(In1)
  Selector2/1 -> syn_gpegpi1/2(In2)
  In4/1 -> Selector5/2, Selector2/2, gpi_cell/4(In4), Selector1/2
  Selector5/1 -> syn_stngpi/2(In2)
  Selector1/1 -> syn_gpegpi/2(In2)
  Constant2/1 -> Selector2/1
  Constant/1 -> Selector5/1
  Constant1/1 -> Selector1/1
  In5/1 -> gpi_cell/5(In5)

== system GPI1/gpicomp6 ==
  In1 : Inport  OutDataType=sfix(16)  OutScaling=2^0
  In2 : Inport  Port=2  OutDataType=sfix(16)  OutScaling=2^0
  In3 : Inport  Port=3  OutDataType=sfix(16)  OutScaling=2^0
  In4 : Inport  Port=4  OutDataType=sfix(16)  OutScaling=2^0
  In5 : Inport  Port=5  OutDataType=sfix(16)  OutScaling=2^0
  Constant : Constant  Value=sis0  OutDataType=sfix(16)  OutScaling=2^0
  Constant1 : Constant  Value=sig0  OutDataType=sfix(16)  OutScaling=2^0
  Constant2 : Constant  Value=sgi0  OutDataType=sfix(16)  OutScaling=2^0
  Selector1 : Selector  IndexMode=Zero-based  IndexOptions=Index vector (port)  Indices=[1 3]  OutputSizes=1
  Selector2 : Selector  IndexMode=Zero-based  IndexOptions=Index vector (port)  Indices=[1 3]  OutputSizes=1
  Selector5 : Selector  IndexMode=Zero-based  IndexOptions=Index vector (port)  Indices=[1 3]  OutputSizes=1
  gpi_cell : Subsystem
  igpegpi : Subsystem
  istngpi : Subsystem
  syn_gpegpi : Subsystem
  syn_gpegpi1 : Subsystem
  syn_stngpi : Subsystem
  Out1 : Outport  OutDataType=sfix(16)  OutScaling=2^0
  Out2 : Outport  Port=2  OutDataType=sfix(16)  OutScaling=2^0
  wires:
  igpegpi/1(Out1) -> gpi_cell/3(In3)
  istngpi/1(Out1) -> gpi_cell/2(In2)
  syn_gpegpi/1(Out1) -> igpegpi/1(In1)
  syn_stngpi/1(Out1) -> istngpi/1(In1)
  syn_gpegpi1/1(Out1) -> Out1/1
  In1/1 -> gpi_cell/1(In1)
  In2/1 -> syn_stngpi/1(In1)
  In3/1 -> syn_gpegpi/1(In1)
  gpi_cell/1(Out1) -> Out2/1, istngpi/2(In3), igpegpi/2(In3), syn_gpegpi1/1(In1)
  Selector2/1 -> syn_gpegpi1/2(In2)
  In4/1 -> Selector5/2, Selector2/2, gpi_cell/4(In4), Selector1/2
  Selector5/1 -> syn_stngpi/2(In2)
  Selector1/1 -> syn_gpegpi/2(In2)
  Constant2/1 -> Selector2/1
  Constant/1 -> Selector5/1
  Constant1/1 -> Selector1/1
  In5/1 -> gpi_cell/5(In5)

== system GPI1/gpicomp7 ==
  In1 : Inport  OutDataType=sfix(16)  OutScaling=2^0
  In2 : Inport  Port=2  OutDataType=sfix(16)  OutScaling=2^0
  In3 : Inport  Port=3  OutDataType=sfix(16)  OutScaling=2^0
  In4 : Inport  Port=4  OutDataType=sfix(16)  OutScaling=2^0
  In5 : Inport  Port=5  OutDataType=sfix(16)  OutScaling=2^0
  Constant : Constant  Value=sis0  OutDataType=sfix(16)  OutScaling=2^0
  Constant1 : Constant  Value=sig0  OutDataType=sfix(16)  OutScaling=2^0
  Constant2 : Constant  Value=sgi0  OutDataType=sfix(16)  OutScaling=2^0
  Selector1 : Selector  IndexMode=Zero-based  IndexOptions=Index vector (port)  Indices=[1 3]  OutputSizes=1
  Selector2 : Selector  IndexMode=Zero-based  IndexOptions=Index vector (port)  Indices=[1 3]  OutputSizes=1
  Selector5 : Selector  IndexMode=Zero-based  IndexOptions=Index vector (port)  Indices=[1 3]  OutputSizes=1
  gpi_cell : Subsystem
  igpegpi : Subsystem
  istngpi : Subsystem
  syn_gpegpi : Subsystem
  syn_gpegpi1 : Subsystem
  syn_stngpi : Subsystem
  Out1 : Outport  OutDataType=sfix(16)  OutScaling=2^0
  Out2 : Outport  Port=2  OutDataType=sfix(16)  OutScaling=2^0
  wires:
  igpegpi/1(Out1) -> gpi_cell/3(In3)
  istngpi/1(Out1) -> gpi_cell/2(In2)
  syn_gpegpi/1(Out1) -> igpegpi/1(In1)
  syn_stngpi/1(Out1) -> istngpi/1(In1)
  syn_gpegpi1/1(Out1) -> Out1/1
  In1/1 -> gpi_cell/1(In1)
  In2/1 -> syn_stngpi/1(In1)
  In3/1 -> syn_gpegpi/1(In1)
  gpi_cell/1(Out1) -> Out2/1, istngpi/2(In3), igpegpi/2(In3), syn_gpegpi1/1(In1)
  Selector2/1 -> syn_gpegpi1/2(In2)
  In4/1 -> Selector5/2, Selector2/2, gpi_cell/4(In4), Selector1/2
  Selector5/1 -> syn_stngpi/2(In2)
  Selector1/1 -> syn_gpegpi/2(In2)
  Constant2/1 -> Selector2/1
  Constant/1 -> Selector5/1
  Constant1/1 -> Selector1/1
  In5/1 -> gpi_cell/5(In5)

== system GPI1/gpicomp8 ==
  In1 : Inport  OutDataType=sfix(16)  OutScaling=2^0
  In2 : Inport  Port=2  OutDataType=sfix(16)  OutScaling=2^0
  In3 : Inport  Port=3  OutDataType=sfix(16)  OutScaling=2^0
  In4 : Inport  Port=4  OutDataType=sfix(16)  OutScaling=2^0
  In5 : Inport  Port=5  OutDataType=sfix(16)  OutScaling=2^0
  Constant : Constant  Value=sis0  OutDataType=sfix(16)  OutScaling=2^0
  Constant1 : Constant  Value=sig0  OutDataType=sfix(16)  OutScaling=2^0
  Constant2 : Constant  Value=sgi0  OutDataType=sfix(16)  OutScaling=2^0
  Selector1 : Selector  IndexMode=Zero-based  IndexOptions=Index vector (port)  Indices=[1 3]  OutputSizes=1
  Selector2 : Selector  IndexMode=Zero-based  IndexOptions=Index vector (port)  Indices=[1 3]  OutputSizes=1
  Selector5 : Selector  IndexMode=Zero-based  IndexOptions=Index vector (port)  Indices=[1 3]  OutputSizes=1
  gpi_cell : Subsystem
  igpegpi : Subsystem
  istngpi : Subsystem
  syn_gpegpi : Subsystem
  syn_gpegpi1 : Subsystem
  syn_stngpi : Subsystem
  Out1 : Outport  OutDataType=sfix(16)  OutScaling=2^0
  Out2 : Outport  Port=2  OutDataType=sfix(16)  OutScaling=2^0
  wires:
  igpegpi/1(Out1) -> gpi_cell/3(In3)
  istngpi/1(Out1) -> gpi_cell/2(In2)
  syn_gpegpi/1(Out1) -> igpegpi/1(In1)
  syn_stngpi/1(Out1) -> istngpi/1(In1)
  syn_gpegpi1/1(Out1) -> Out1/1
  In1/1 -> gpi_cell/1(In1)
  In2/1 -> syn_stngpi/1(In1)
  In3/1 -> syn_gpegpi/1(In1)
  gpi_cell/1(Out1) -> Out2/1, istngpi/2(In3), igpegpi/2(In3), syn_gpegpi1/1(In1)
  Selector2/1 -> syn_gpegpi1/2(In2)
  In4/1 -> Selector5/2, Selector2/2, gpi_cell/4(In4), Selector1/2
  Selector5/1 -> syn_stngpi/2(In2)
  Selector1/1 -> syn_gpegpi/2(In2)
  Constant2/1 -> Selector2/1
  Constant/1 -> Selector5/1
  Constant1/1 -> Selector1/1
  In5/1 -> gpi_cell/5(In5)

== system GPI1/gpicomp9 ==
  In1 : Inport  OutDataType=sfix(16)  OutScaling=2^0
  In2 : Inport  Port=2  OutDataType=sfix(16)  OutScaling=2^0
  In3 : Inport  Port=3  OutDataType=sfix(16)  OutScaling=2^0
  In4 : Inport  Port=4  OutDataType=sfix(16)  OutScaling=2^0
  In5 : Inport  Port=5  OutDataType=sfix(16)  OutScaling=2^0
  Constant : Constant  Value=sis0  OutDataType=sfix(16)  OutScaling=2^0
  Constant1 : Constant  Value=sig0  OutDataType=sfix(16)  OutScaling=2^0
  Constant2 : Constant  Value=sgi0  OutDataType=sfix(16)  OutScaling=2^0
  Selector1 : Selector  IndexMode=Zero-based  IndexOptions=Index vector (port)  Indices=[1 3]  OutputSizes=1
  Selector2 : Selector  IndexMode=Zero-based  IndexOptions=Index vector (port)  Indices=[1 3]  OutputSizes=1
  Selector5 : Selector  IndexMode=Zero-based  IndexOptions=Index vector (port)  Indices=[1 3]  OutputSizes=1
  gpi_cell : Subsystem
  igpegpi : Subsystem
  istngpi : Subsystem
  syn_gpegpi : Subsystem
  syn_gpegpi1 : Subsystem
  syn_stngpi : Subsystem
  Out1 : Outport  OutDataType=sfix(16)  OutScaling=2^0
  Out2 : Outport  Port=2  OutDataType=sfix(16)  OutScaling=2^0
  wires:
  igpegpi/1(Out1) -> gpi_cell/3(In3)
  istngpi/1(Out1) -> gpi_cell/2(In2)
  syn_gpegpi/1(Out1) -> igpegpi/1(In1)
  syn_stngpi/1(Out1) -> istngpi/1(In1)
  syn_gpegpi1/1(Out1) -> Out1/1
  In1/1 -> gpi_cell/1(In1)
  In2/1 -> syn_stngpi/1(In1)
  In3/1 -> syn_gpegpi/1(In1)
  gpi_cell/1(Out1) -> Out2/1, istngpi/2(In3), igpegpi/2(In3), syn_gpegpi1/1(In1)
  Selector2/1 -> syn_gpegpi1/2(In2)
  In4/1 -> Selector5/2, Selector2/2, gpi_cell/4(In4), Selector1/2
  Selector5/1 -> syn_stngpi/2(In2)
  Selector1/1 -> syn_gpegpi/2(In2)
  Constant2/1 -> Selector2/1
  Constant/1 -> Selector5/1
  Constant1/1 -> Selector1/1
  In5/1 -> gpi_cell/5(In5)

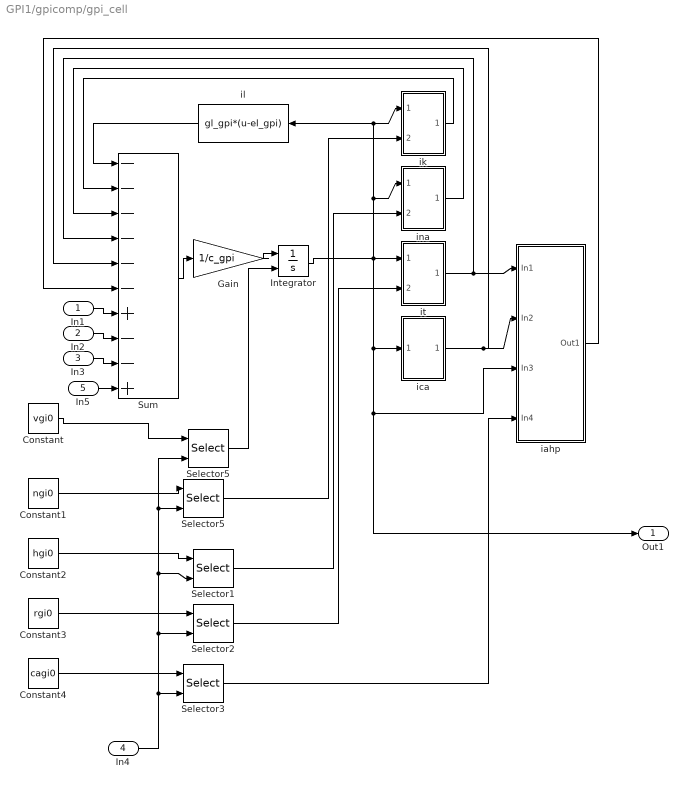
== system GPI1/gpicomp/gpi_cell ==
  In1 : Inport  OutDataType=sfix(16)  OutScaling=2^0
  In2 : Inport  Port=2  OutDataType=sfix(16)  OutScaling=2^0
  In3 : Inport  Port=3  OutDataType=sfix(16)  OutScaling=2^0
  In4 : Inport  Port=4  OutDataType=sfix(16)  OutScaling=2^0
  In5 : Inport  Port=5  OutDataType=sfix(16)  OutScaling=2^0
  Constant : Constant  Value=vgi0  OutDataType=sfix(16)  OutScaling=2^0
  Constant1 : Constant  Value=ngi0  OutDataType=sfix(16)  OutScaling=2^0
  Constant2 : Constant  Value=hgi0  OutDataType=sfix(16)  OutScaling=2^0
  Constant3 : Constant  Value=rgi0  OutDataType=sfix(16)  OutScaling=2^0
  Constant4 : Constant  Value=cagi0  OutDataType=sfix(16)  OutScaling=2^0
  Gain : Gain  Gain=1/c_gpi  ParameterDataType=sfix(16)  ParameterScaling=2^0  OutDataType=sfix(16)  OutScaling=2^0  SaturateOnIntegerOverflow=on
  Integrator : Integrator  InitialConditionSource=external  InitialCondition=-67  LimitOutput=on  UpperSaturationLimit=80
  Selector{1..3,5} (4 alike) : Selector  IndexMode=Zero-based  IndexOptions=Index vector (port)  Indices=[1 3]  OutputSizes=1
  "Selector5 " : Selector  IndexMode=Zero-based  IndexOptions=Index vector (port)  Indices=[1 3]  OutputSizes=1
  Sum : Sum  Description=--------  Inputs=------+--+  OutDataType=sfix(16)  OutScaling=2^0  SaturateOnIntegerOverflow=on  InputSameDT=on
  iahp : Subsystem
  ica : Subsystem
  ik : Subsystem
  il : Fcn  Orientation=left  Expr=gl_gpi*(u-el_gpi)
  ina : Subsystem
  it : Subsystem
  Out1 : Outport  OutDataType=sfix(16)  OutScaling=2^0
  wires:
  Gain/1 -> Integrator/1
  Sum/1 -> Gain/1
  Integrator/1 -> il/1, ik/1(In1), ina/1(In2), it/1(In2), ica/1(In1), iahp/3(In3), Out1/1
  il/1 -> Sum/1
  ik/1(Out1) -> Sum/2
  ina/1(Out1) -> Sum/3
  ica/1(Out1) -> iahp/2(In2), Sum/5
  it/1(Out1) -> iahp/1(In1), Sum/4
  iahp/1(Out1) -> Sum/6
  In1/1 -> Sum/7
  In2/1 -> Sum/8
  In3/1 -> Sum/9
  "Selector5 "/1 -> Integrator/2
  Selector5/1 -> ik/2(In2)
  Selector1/1 -> ina/2(In1)
  Selector2/1 -> it/2(In1)
  Selector3/1 -> iahp/4(In4)
  In4/1 -> "Selector5 "/2, Selector5/2, Selector1/2, Selector2/2, Selector3/2
  Constant/1 -> "Selector5 "/1
  Constant1/1 -> Selector5/1
  Constant2/1 -> Selector1/1
  Constant3/1 -> Selector2/1
  Constant4/1 -> Selector3/1
  In5/1 -> Sum/10

== system GPI1/gpicomp/igpegpi ==
  In1 : Inport  OutDataType=sfix(16)  OutScaling=2^0
  In3 : Inport  Port=2  OutDataType=sfix(16)  OutScaling=2^0
  Fcn : Fcn  Expr=ggpegpi*(u-egpegpi)
  Product : Product  OutDataType=sfix(16)  OutScaling=2^0  SaturateOnIntegerOverflow=on  InputSameDT=on
  Out1 : Outport  OutDataType=sfix(16)  OutScaling=2^0
  wires:
  Fcn/1 -> Product/2
  In1/1 -> Product/1
  Product/1 -> Out1/1
  In3/1 -> Fcn/1

== system GPI1/gpicomp/istngpi ==
  In1 : Inport  OutDataType=sfix(16)  OutScaling=2^0
  In3 : Inport  Port=2  OutDataType=sfix(16)  OutScaling=2^0
  Fcn : Fcn  Expr=gstngpi*(u-estngpi)
  Product : Product  OutDataType=sfix(16)  OutScaling=2^0  SaturateOnIntegerOverflow=on  InputSameDT=on
  Out1 : Outport  OutDataType=sfix(16)  OutScaling=2^0
  wires:
  Fcn/1 -> Product/2
  In1/1 -> Product/1
  Product/1 -> Out1/1
  In3/1 -> Fcn/1

== system GPI1/gpicomp/syn_gpegpi ==
  In1 : Inport  OutDataType=sfix(16)  OutScaling=2^0
  In2 : Inport  Port=2  OutDataType=sfix(16)  OutScaling=2^0
  Fcn : Fcn  Expr=1/(1+exp(-(u-theta_gpe-thetagh_gpe)/sigmagh_gpe))
  Fcn2 : Fcn  Orientation=left  Expr=A_gpegpi*(1-u)
  Gain : Gain  Orientation=left  Gain=B_gpegpi  ParameterDataType=sfix(16)  ParameterScaling=2^0  OutDataType=sfix(16)  OutScaling=2^0  SaturateOnIntegerOverflow=on
  Integrator : Integrator  InitialConditionSource=external
  Product : Product  OutDataType=sfix(16)  OutScaling=2^0  SaturateOnIntegerOverflow=on  InputSameDT=on
  Sum : Sum  Inputs=|+-  OutDataType=sfix(16)  OutScaling=2^0  SaturateOnIntegerOverflow=on  InputSameDT=on
  Out1 : Outport  OutDataType=sfix(16)  OutScaling=2^0
  wires:
  Fcn/1 -> Product/1
  Fcn2/1 -> Product/2
  Product/1 -> Sum/1
  Sum/1 -> Integrator/1
  Integrator/1 -> Gain/1, Fcn2/1, Out1/1
  Gain/1 -> Sum/2
  In1/1 -> Fcn/1
  In2/1 -> Integrator/2

== system GPI1/gpicomp/syn_gpegpi1 ==
  In1 : Inport  OutDataType=sfix(16)  OutScaling=2^0
  In2 : Inport  Port=2  OutDataType=sfix(16)  OutScaling=2^0
  Fcn : Fcn  Expr=1/(1+exp(-(u-theta_gpi-thetagh_gpi)/sigmagh_gpi))
  Fcn2 : Fcn  Orientation=left  Expr=A_gpi*(1-u)
  Gain : Gain  Orientation=left  Gain=B_gpi  ParameterDataType=sfix(16)  ParameterScaling=2^0  OutDataType=sfix(16)  OutScaling=2^0  SaturateOnIntegerOverflow=on
  Integrator : Integrator  InitialConditionSource=external
  Product : Product  OutDataType=sfix(16)  OutScaling=2^0  SaturateOnIntegerOverflow=on  InputSameDT=on
  Sum : Sum  Inputs=|+-  OutDataType=sfix(16)  OutScaling=2^0  SaturateOnIntegerOverflow=on  InputSameDT=on
  Out1 : Outport  OutDataType=sfix(16)  OutScaling=2^0
  wires:
  Fcn/1 -> Product/1
  Fcn2/1 -> Product/2
  Product/1 -> Sum/1
  Sum/1 -> Integrator/1
  Integrator/1 -> Gain/1, Fcn2/1, Out1/1
  Gain/1 -> Sum/2
  In1/1 -> Fcn/1
  In2/1 -> Integrator/2

== system GPI1/gpicomp/syn_stngpi ==
  In1 : Inport  OutDataType=sfix(16)  OutScaling=2^0
  In2 : Inport  Port=2  OutDataType=sfix(16)  OutScaling=2^0
  Fcn : Fcn  Expr=1/(1+exp(-(u-theta_stn-thetagh_stn)/sigmagh_stn))
  Fcn2 : Fcn  Orientation=left  Expr=A_stngpi*(1-u)
  Gain : Gain  Orientation=left  Gain=B_stngpi  ParameterDataType=sfix(16)  ParameterScaling=2^0  OutDataType=sfix(16)  OutScaling=2^0  SaturateOnIntegerOverflow=on
  Integrator : Integrator  InitialConditionSource=external
  Product : Product  OutDataType=sfix(16)  OutScaling=2^0  SaturateOnIntegerOverflow=on  InputSameDT=on
  Sum : Sum  Inputs=|+-  OutDataType=sfix(16)  OutScaling=2^0  SaturateOnIntegerOverflow=on  InputSameDT=on
  Out1 : Outport  OutDataType=sfix(16)  OutScaling=2^0
  wires:
  Fcn/1 -> Product/1
  Fcn2/1 -> Product/2
  Product/1 -> Sum/1
  Sum/1 -> Integrator/1
  Integrator/1 -> Gain/1, Fcn2/1, Out1/1
  Gain/1 -> Sum/2
  In1/1 -> Fcn/1
  In2/1 -> Integrator/2

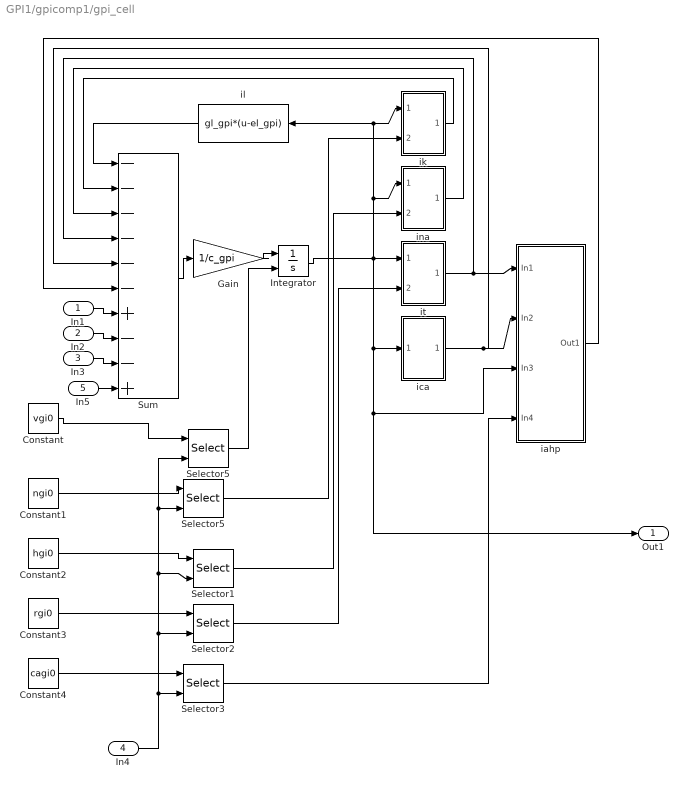
== system GPI1/gpicomp1/gpi_cell ==
  In1 : Inport  OutDataType=sfix(16)  OutScaling=2^0
  In2 : Inport  Port=2  OutDataType=sfix(16)  OutScaling=2^0
  In3 : Inport  Port=3  OutDataType=sfix(16)  OutScaling=2^0
  In4 : Inport  Port=4  OutDataType=sfix(16)  OutScaling=2^0
  In5 : Inport  Port=5  OutDataType=sfix(16)  OutScaling=2^0
  Constant : Constant  Value=vgi0  OutDataType=sfix(16)  OutScaling=2^0
  Constant1 : Constant  Value=ngi0  OutDataType=sfix(16)  OutScaling=2^0
  Constant2 : Constant  Value=hgi0  OutDataType=sfix(16)  OutScaling=2^0
  Constant3 : Constant  Value=rgi0  OutDataType=sfix(16)  OutScaling=2^0
  Constant4 : Constant  Value=cagi0  OutDataType=sfix(16)  OutScaling=2^0
  Gain : Gain  Gain=1/c_gpi  ParameterDataType=sfix(16)  ParameterScaling=2^0  OutDataType=sfix(16)  OutScaling=2^0  SaturateOnIntegerOverflow=on
  Integrator : Integrator  InitialConditionSource=external  InitialCondition=-67  LimitOutput=on  UpperSaturationLimit=80
  Selector{1..3,5} (4 alike) : Selector  IndexMode=Zero-based  IndexOptions=Index vector (port)  Indices=[1 3]  OutputSizes=1
  "Selector5 " : Selector  IndexMode=Zero-based  IndexOptions=Index vector (port)  Indices=[1 3]  OutputSizes=1
  Sum : Sum  Description=--------  Inputs=------+--+  OutDataType=sfix(16)  OutScaling=2^0  SaturateOnIntegerOverflow=on  InputSameDT=on
  iahp : Subsystem
  ica : Subsystem
  ik : Subsystem
  il : Fcn  Orientation=left  Expr=gl_gpi*(u-el_gpi)
  ina : Subsystem
  it : Subsystem
  Out1 : Outport  OutDataType=sfix(16)  OutScaling=2^0
  wires:
  Gain/1 -> Integrator/1
  Sum/1 -> Gain/1
  Integrator/1 -> il/1, ik/1(In1), ina/1(In2), it/1(In2), ica/1(In1), iahp/3(In3), Out1/1
  il/1 -> Sum/1
  ik/1(Out1) -> Sum/2
  ina/1(Out1) -> Sum/3
  ica/1(Out1) -> iahp/2(In2), Sum/5
  it/1(Out1) -> iahp/1(In1), Sum/4
  iahp/1(Out1) -> Sum/6
  In1/1 -> Sum/7
  In2/1 -> Sum/8
  In3/1 -> Sum/9
  "Selector5 "/1 -> Integrator/2
  Selector5/1 -> ik/2(In2)
  Selector1/1 -> ina/2(In1)
  Selector2/1 -> it/2(In1)
  Selector3/1 -> iahp/4(In4)
  In4/1 -> "Selector5 "/2, Selector5/2, Selector1/2, Selector2/2, Selector3/2
  Constant/1 -> "Selector5 "/1
  Constant1/1 -> Selector5/1
  Constant2/1 -> Selector1/1
  Constant3/1 -> Selector2/1
  Constant4/1 -> Selector3/1
  In5/1 -> Sum/10

== system GPI1/gpicomp1/igpegpi ==
  In1 : Inport  OutDataType=sfix(16)  OutScaling=2^0
  In3 : Inport  Port=2  OutDataType=sfix(16)  OutScaling=2^0
  Fcn : Fcn  Expr=ggpegpi*(u-egpegpi)
  Product : Product  OutDataType=sfix(16)  OutScaling=2^0  SaturateOnIntegerOverflow=on  InputSameDT=on
  Out1 : Outport  OutDataType=sfix(16)  OutScaling=2^0
  wires:
  Fcn/1 -> Product/2
  In1/1 -> Product/1
  Product/1 -> Out1/1
  In3/1 -> Fcn/1

== system GPI1/gpicomp1/istngpi ==
  In1 : Inport  OutDataType=sfix(16)  OutScaling=2^0
  In3 : Inport  Port=2  OutDataType=sfix(16)  OutScaling=2^0
  Fcn : Fcn  Expr=gstngpi*(u-estngpi)
  Product : Product  OutDataType=sfix(16)  OutScaling=2^0  SaturateOnIntegerOverflow=on  InputSameDT=on
  Out1 : Outport  OutDataType=sfix(16)  OutScaling=2^0
  wires:
  Fcn/1 -> Product/2
  In1/1 -> Product/1
  Product/1 -> Out1/1
  In3/1 -> Fcn/1
